simulink model "Copy_of_Reaching"  (R2023b)
settings: Solver=FixedStepDiscrete  StartTime=0.0  StopTime=inf  FixedStep=0.001  RelTol=1e-3
libraries: vrlib x1
settings Model: Creator=carlos.aldana  LastModifiedBy=miryr
settings SolverCC: AlgebraicLoopSolver=TrustRegion
settings DataIOCC: LimitDataPoints=on  SaveFormat=Array  ReturnWorkspaceOutputs=off
settings OptimizationCC: BlockReduction=off  BooleanDataType=off  LifeSpan=inf
settings DebuggingCC: SaveWithParameterizedLinksMsg=none  UnderspecifiedInitializationDetection=Classic  MergeDetectMultiDrivingBlocksExec=none  SignalResolutionControl=TryResolveAllWithWarning  UnconnectedInputMsg=warning  UnconnectedOutputMsg=warning  UnconnectedLineMsg=warning  AllowSymbolicDim=off  SFUnexpectedBacktrackingDiag=warning  SFNoUnconditionalDefaultTransitionDiag=warning  SFExecutionAtInitializationDiag=none  ArithmeticOperatorsInVariantConditions=warning
settings HardwareCC: ProdBitPerPointer=32  ProdBitPerSizeT=32  ProdBitPerPtrDiffT=32  ProdLargestAtomicFloat=None  ProdIntDivRoundTo=Undefined  ProdEndianess=Unspecified  ProdWordSize=32  ProdHWDeviceType=32-bit Generic  TargetUnknown=on
settings ModelReferenceCC: EnableRefExpFcnMdlSchedulingChecks=on  PropagateSignalLabelsOutOfModel=off
settings SFSimCC: SimUseLocalCustomCode=off  CustomCodeUndefinedFunction=UseInterfaceOnly
settings RTWCC: RTWUseLocalCustomCode=off  DLArmComputeVersion=19.05
settings CodeAppCC: StateflowObjectComments=on
settings GRTTargetCC: TargetLangStandard=C89/C90 (ANSI)
settings ConfigComp: CovMetricSettings=dw  CovSaveCumulativeToWorkspaceVar=on  CovSaveSingleToWorkspaceVar=on  CovExternalEMLEnable=off  CovSFcnEnable=off

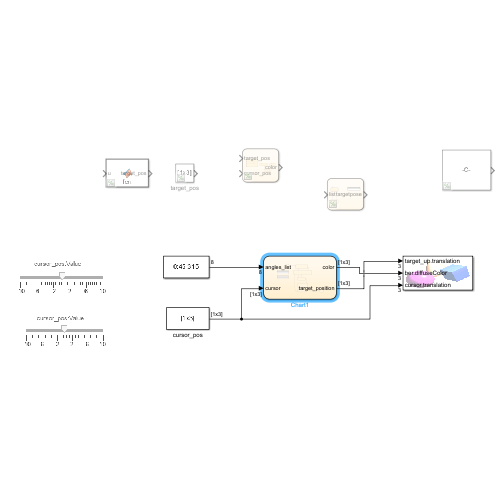
[thumbnail: Simulink's stored preview of the top-level diagram]
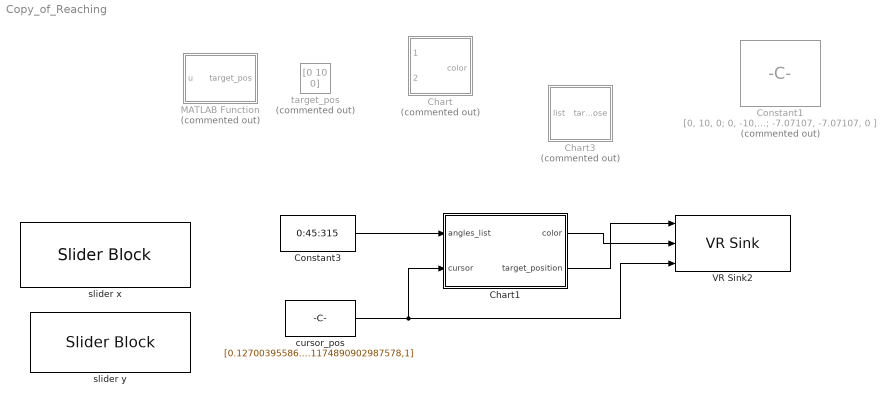
== system Copy_of_Reaching ==
  Chart : Stateflow chart  Commented=on  TreatAsAtomicUnit=on
  Chart1 : Stateflow chart  TreatAsAtomicUnit=on
  Chart3 : Stateflow chart  Commented=on  TreatAsAtomicUnit=on
  Constant1 : Constant  Commented=on  Value=|
      | [0, 10, 0;
      | 0, -10, 0;
      | 10, 0, 0;
      | -10, 0, 0; 7.07107, 7.07107, 0;
      | -7.07107, 7.07107, 0;
      | 7.07107, -7.07107, 0; -7.07107, -7.07107, 0
      | ]
  Constant3 : Constant  Value=0:45:315
  MATLAB Function : MATLAB Function  Commented=on  TreatAsAtomicUnit=on
  VR Sink2 : vrlib/VR Sink  InstantiateOnLoad=on  SampleTime=0.01  ViewEnable=on  RemoteChange=off  RemoteView=off  FieldsWritten=target_up.translation.3.1.1.double#ber.diffuseColor.3.1.1.double#cursor.translation.3.1.1.double  WorldFileName=2_palline_color.wrl  AutoView=off  VideoDimensions=[]  AllowVariableSize=off
  cursor_pos : Constant  Value=[0.1270039558609213,-0.1174890902987578,1]  VectorParams1D=off
  slider x : SliderBlock  ScaleMin=-10  ScaleMax=10
  slider y : SliderBlock  ScaleMin=-10  ScaleMax=10
  target_pos : Constant  Commented=on  Value=[0 10 0]
  wires:
  Chart1/1(color) -> VR Sink2/2
  cursor_pos/1 -> VR Sink2/3, Chart1/2(cursor)
  Constant3/1 -> Chart1/1(angles_list)
  Chart1/2(target_position) -> VR Sink2/1

== matlab function Copy_of_Reaching/MATLAB Function ==
  data: u input; target_pos output
function target_pos = fcn(u)

% Numero totale di coordinate
num_coordinate = size(u, 1);

% Scegli casualmente una coordinata senza ripetersi
indici_casuali = randperm(num_coordinate);

for i = 1:num_coordinate
    % Ottieni l'indice casuale corrente
    indice_scelto = indici_casuali(i);
    
    % Ottieni la coordinata corrispondente all'indice scelto
    target_pos = u(indice_scelto, :);

    pause(0.2);
end

== stateflow chart Copy_of_Reaching/Chart ==
  state c = check_center(cur, tar) [function]
    (default) -> (junction 22) : % check the center
    (junction 22) -> (junction 23) [order 1] : [abs(tar(2) - cur(2)) <= 0.2]
    (junction 22) -> (junction 24) [order 2] : {c = [0.1 0.6 1];}
    (junction 23) -> (junction 25) : {c = [0 0.8 1];}
    (junction 25) -> (junction 24)
    (junction 24) -> (junction 26)
  state Reaching1
    entry:
    c = cursor_pos;
  state Reaching2
    entry:
    t = target_pos;
  state reach
    during:
    color = check_center(c, t);
  (default) -> Reaching1 [order 1] : [cursor_pos]
  (default) -> Reaching2 [order 2] : [target_pos]
  Reaching2 -> reach
  Reaching1 -> reach
  data: cur function_input; c function_output; tar function_input; target_pos input; cursor_pos input; color output; c local; t local

== stateflow chart Copy_of_Reaching/Chart3 ==
  state onstart
    targetpose=list(1, :);
  state During
    targetpose=[0 0 0];
  (default) -> onstart : list
  onstart -> During : after(10,sec)
  During -> onstart : after(10,sec)
  data: u function_input; target_pos function_output; targetpose output; list input
  function target_pos = fcn(u):
    | function target_pos = fcn(u)
    | 
    | % Numero totale di coordinate
    | num_coordinate = size(u, 1);
    | 
    | % Scegli casualmente una coordinata senza ripetersi
    | indici_casuali = randperm(num_coordinate);
    | 
    | 
    | 
    |     
    | % Ottieni la coordinata corrispondente all'indice scelto
    | target_pos = u(indici_casuali, 1);
    | 
    | pause(0.2);

== stateflow chart Copy_of_Reaching/Chart1 ==
  state StartState
    entry:
    i=1;
  state RandomAngleGeneration
    entry:
    random_angles_list = randomAngle(angles_list);
    idx = 1;
  state ShowTarget
    entry:
    color = [1 0.2 0.2];
    target_position = computeTargetPose(random_angles_list(idx));
  state ReachingColor
    entry:
    color = [0 0.8 1];
  state ChnageTargetPosition
    entry:
    target_position = [0 0 0];
    color = [1 0.2 0.2];
  state finishState
    color=[0 0.5 0];
  state ReachingColor1
    entry:
    color = [0 0.8 1];
  (default) -> StartState [order 1]
  (default) -> StartState [order 2]
  StartState -> RandomAngleGeneration
  ShowTarget -> RandomAngleGeneration [order 2] : [idx==8]{i=i+1}
  RandomAngleGeneration -> ShowTarget
  ReachingColor1 -> ShowTarget [order 2] : after(2, sec)[sqrt((target_position(1)-cursor(1))^2 + (target_position(2)-cursor(2))^2) <= 0.2 & i<2]{idx = idx + 1}
  ShowTarget -> ReachingColor [order 1] : [sqrt((target_position(1)-cursor(1))^2 + (target_position(2)-cursor(2))^2) <= 0.2]
  ReachingColor -> ShowTarget [order 1] : [sqrt((target_position(1)-cursor(1))^2 + (target_position(2)-cursor(2))^2) > 0.2]
  ReachingColor -> ChnageTargetPosition [order 2] : after(2, sec)[sqrt((target_position(1)-cursor(1))^2 + (target_position(2)-cursor(2))^2) <= 0.2]
  ChnageTargetPosition -> ReachingColor1 : [sqrt((target_position(1)-cursor(1))^2 + (target_position(2)-cursor(2))^2) <= 0.2]
  ReachingColor1 -> ChnageTargetPosition [order 1] : [sqrt((target_position(1)-cursor(1))^2 + (target_position(2)-cursor(2))^2) > 0.2]
  ReachingColor1 -> finishState [order 3] : [idx==2 &i==2]
  data: al function_input; random_list function_output; angle function_input; r function_output; color output; angles_list input; cursor input; target_position output; idx local; random_angles_list local; i local
  function random_list = randomAngle(al):
    | function random_list = randomAngle(al)
    |     size_list = length(al);
    |     random_index = randperm(size_list);
    |     
    |     % Inizializza la nuova lista con le stesse dimensioni di al
    |     new_list = zeros(size_list, 1);
    | 
    |     for i = 1:size_list
    |         % Assegna gli elementi di al nell'ordine casuale
    |         new_list(i) = al(random_index(i));
    |     end
    | 
    |     random_list = new_list;
    | end
  function r = computeTargetPose(angle):
    | function r = computeTargetPose(angle)
    |     % Converti l'angolo da gradi a radianti
    |     theta = deg2rad(angle);
    | 
    |     % Calcola le coordinate del punto sulla circonferenza
    |     x = 10 * cos(theta);
    |     y = 10 * sin(theta);
    |     z = 0;
    |     r =[x y z];
    | end
